simulink model "Pendulum_model_linid"  (R2016a)
settings: Solver=ode45  StartTime=0.0  StopTime=10  RelTol=1e-3
model workspace: external: MATLAB File D:\Documenten\Biomedical Engineering\2016-2017\Control Systems Lab\Lab sessie 1\CSL\Dick\params.m (data not in the file)
values from neighbouring files (symbols this model uses):
  h = 0.01    [Pendulum_linid.m]    (also in draw_pendulum.m = plot(0,0,'MarkerSize',20,'Marker','+','LineWidth',5); linid.m = 0.1; params.m)
  k_m = 50    [linearization_by_hand.m]    (also in params.m = 41.0587; symbolic_derivation.m)
  tau_e = 0.03    [linearization_by_hand.m]    (also in params.m = 0.0312; symbolic_derivation.m)
  u0 = 0    [Pendulum_linid.m]
  x0 = [pi;0;0;0;0]    [Pendulum_linid.m]    (also in linid.m = [2;0])
settings Model: Creator=Nathan  LastModifiedBy=Dick
settings DataIOCC: InitialState=states  LimitDataPoints=on  LoadInitialState=on  SaveFormat=Array
settings DebuggingCC: AllowSymbolicDim=off
settings HardwareCC: ProdBitPerPointer=32  ProdLargestAtomicFloat=None  ProdIntDivRoundTo=Undefined  ProdEndianess=Unspecified  ProdWordSize=32  ProdHWDeviceType=32-bit Generic
settings ModelReferenceCC: PropagateSignalLabelsOutOfModel=off
settings ConfigComp: CovModelRefEnable=Off

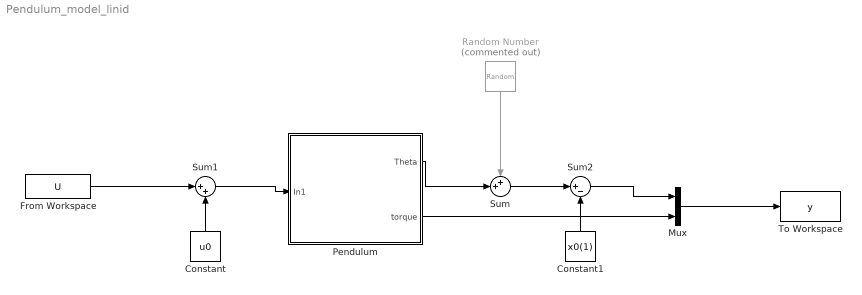
== system Pendulum_model_linid ==
  Constant : Constant  Value=u0
  Constant1 : Constant  Value=x0(1)
  From Workspace : FromWorkspace  VariableName=U  SampleTime=h
  Mux : Mux  Inputs=2
  Pendulum : Subsystem
  Random Number : RandomNumber  Commented=on  Variance=1e-7  SampleTime=h
  Sum : Sum  Inputs=++|
  Sum1 : Sum  Inputs=|++  SaturateOnIntegerOverflow=on  InputSameDT=on  OutDataTypeStr=Inherit: Same as first input
  Sum2 : Sum  Inputs=|+-  SaturateOnIntegerOverflow=on  InputSameDT=on  OutDataTypeStr=Inherit: Same as first input
  To Workspace : ToWorkspace  VariableName=y  SaveFormat=Timeseries  SampleTime=h
  wires:
  Random Number/1 -> Sum/1
  Pendulum/1(Theta) -> Sum/2
  Constant/1 -> Sum1/2
  From Workspace/1 -> Sum1/1
  Sum1/1 -> Pendulum/1(In1)
  Constant1/1 -> Sum2/2
  Sum/1 -> Sum2/1
  Pendulum/2(torque) -> Mux/2
  Sum2/1 -> Mux/1
  Mux/1 -> To Workspace/1

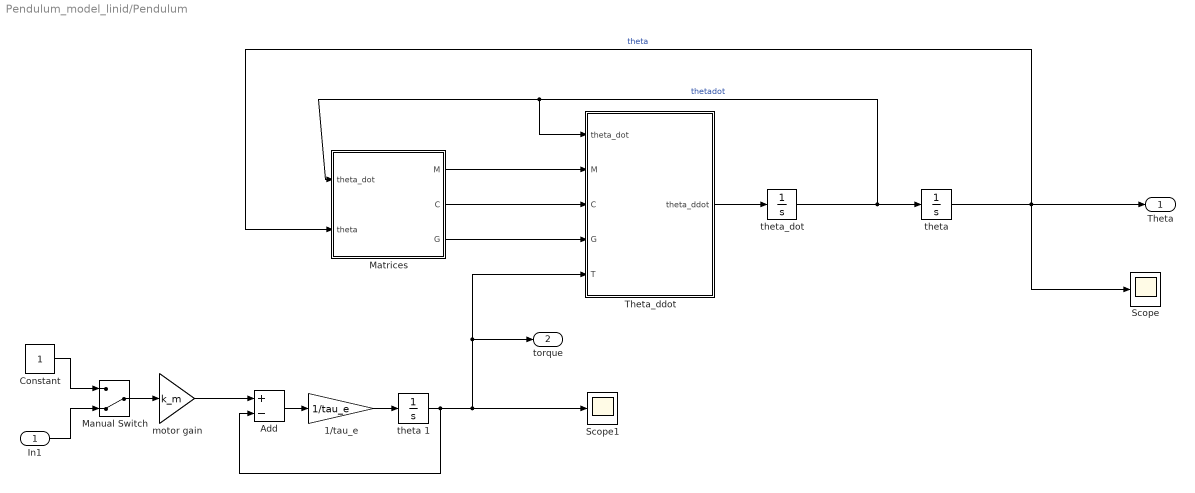
== system Pendulum_model_linid/Pendulum ==
  In1 : Inport
  "1/tau_e " : Gain  Gain=1/tau_e
  Add : Sum  Inputs=+-
  Constant : Constant
  Manual Switch : ManualSwitch  CurrentSetting=0
  Matrices : MATLAB Function  TreatAsAtomicUnit=on
  Scope : Scope
  Scope1 : Scope
  "Theta_ddot " : MATLAB Function  TreatAsAtomicUnit=on
  "motor gain " : Gain  Gain=k_m
  "theta " : Integrator
  theta 1 : Integrator
  "theta_dot " : Integrator
  Theta : Outport
  torque : Outport  Port=2
  wires:
  Manual Switch/1 -> "motor gain "/1
  theta 1/1 -> Add/2, "Theta_ddot "/5(T), torque/1, Scope1/1
  "1/tau_e "/1 -> theta 1/1
  Add/1 -> "1/tau_e "/1
  "motor gain "/1 -> Add/1
  "theta "/1 -> Theta/1, Scope/1, Matrices/2(theta)  "theta"
  "theta_dot "/1 -> "theta "/1, "Theta_ddot "/1(theta_dot), Matrices/1(theta_dot)  "thetadot"
  "Theta_ddot "/1(theta_ddot) -> "theta_dot "/1
  Matrices/3(G) -> "Theta_ddot "/4(G)
  Matrices/2(C) -> "Theta_ddot "/3(C)
  Matrices/1(M) -> "Theta_ddot "/2(M)
  Constant/1 -> Manual Switch/1
  In1/1 -> Manual Switch/2

== matlab function Pendulum_model_linid/Pendulum/Theta_ddot  ==
  data: theta_dot input; M input; C input; G input; theta_ddot output; T input
function theta_ddot = fcn(theta_dot,M,C,G,T)
theta_ddot = [0;0];

theta_ddot = M\[T;0] - M\C*theta_dot - M\G;

== matlab function Pendulum_model_linid/Pendulum/Matrices ==
  data: theta_dot input; theta input; M output; C output; G output
function [M, C, G] = fcn(theta_dot, theta)

M = zeros(2);
C = zeros(2);
G = [0;0];

g = 9.81; 
l1 = 0.1;
l2 = 0.1;
m1 = 0.125;
m2 = 0.05;
c1 = 0.04; % Keeping it negative results in no motion at all, -0.04 or + 0.04?
c2 = 0.06;
I1 = 0.074;
I2 = 0.00012;
b1 = 4.8;
b2 = 0.0002;

P1 = m1*c1^2+m2*l1^2+I1;
P2 = m2*c2^2+ I2;
P3 = m2*l1*c2;
g1 = (m1*c1+m2*l1)*g;
g2 = m2*c2*g;

M = [(P1 + P2 + 2*P3*cos(theta(2)))               (P2 + P3*cos(theta(2))) ;
     (P2 + P3*cos(theta(2)))                       P2                   ];
 
 
C = [(b1 - P3*theta_dot(2)*sin(theta(2)))           (-P3*(theta_dot(1)+theta_dot(2))*sin(theta(2))) ;
     (P3*theta_dot(1)*sin(theta(2)))                 b2                                      ];
     
G = [(-g1*sin(theta(1))-g2*sin(theta(1) + theta(2))) ;
      -g2*sin(theta(1)+theta(2))                   ];
